simulink model "example7_13"  (R2016b)
settings: Solver=VariableStepAuto  StartTime=0.0  StopTime=1  RelTol=1e-3
libraries: dspsrcs4 x2
settings Model: Creator=zhangjin  LastModifiedBy=zhangjin

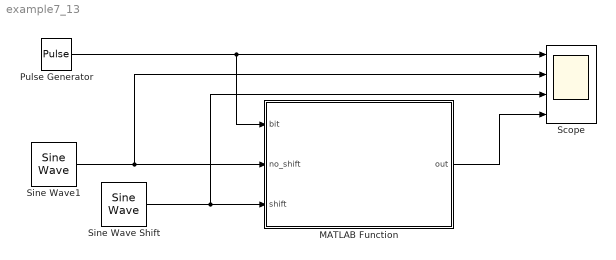
== system example7_13 ==
  MATLAB Function : MATLAB Function  TreatAsAtomicUnit=on
  Pulse Generator : DiscretePulseGenerator  PulseType=Time based  Period=0.2  PulseWidth=50
  Scope : Scope  NumInputPorts=4
  Sine Wave Shift : dspsrcs4/Sine Wave  Amplitude=1  Frequency=10  Phase=pi  SampleMode=Discrete  OutComplex=Real  CompMethod=Trigonometric fcn  TableSize=Speed  SampleTime=1/2000  SamplesPerFrame=1  ResetState=Restart at time zero  OutputFrames=off  dataType=double  wordLen=16  udDataType=sfix(16)  fracBitsMode=Best precision  numFracBits=15  OutDataTypeStr=double  LastOutDataTypeStr=double
  Sine Wave1 : dspsrcs4/Sine Wave  Amplitude=1  Frequency=10  Phase=0  SampleMode=Discrete  OutComplex=Real  CompMethod=Trigonometric fcn  TableSize=Speed  SampleTime=1/2000  SamplesPerFrame=1  ResetState=Restart at time zero  OutputFrames=off  dataType=double  wordLen=16  udDataType=sfix(16)  fracBitsMode=Best precision  numFracBits=15  OutDataTypeStr=double  LastOutDataTypeStr=double
  wires:
  Pulse Generator/1 -> MATLAB Function/1(bit), Scope/1
  Sine Wave1/1 -> Scope/2, MATLAB Function/2(no_shift)
  Sine Wave Shift/1 -> Scope/3, MATLAB Function/3(shift)
  MATLAB Function/1(out) -> Scope/4

== matlab function example7_13/MATLAB Function ==
  data: bit input; out output; no_shift input; shift input

function out =BPSK (bit,no_shift,shift)
if bit == 1
    out = no_shift
else
    out = shift
          end
